simulink model "TITO_OC_2018"  (Simulink 9.1)
settings: Solver=ode45  StartTime=0.0  StopTime=100  RelTol=1e-3  EnableMultiTasking=on
undefined symbols (not defined in the file): T0
libraries: simulink x4
settings Model: Creator=petr  LastModifiedBy=NICHOLAS ANG
settings DataIOCC: LimitDataPoints=on  SignalLoggingSaveFormat=ModelDataLogs
settings OptimizationCC: ExpressionDepthLimit=2147483647  InitFltsAndDblsToZero=on
settings DebuggingCC: SolverPrmCheckMsg=warning  FcnCallInpInsideContextMsg=warning  StateNameClashWarn=warning

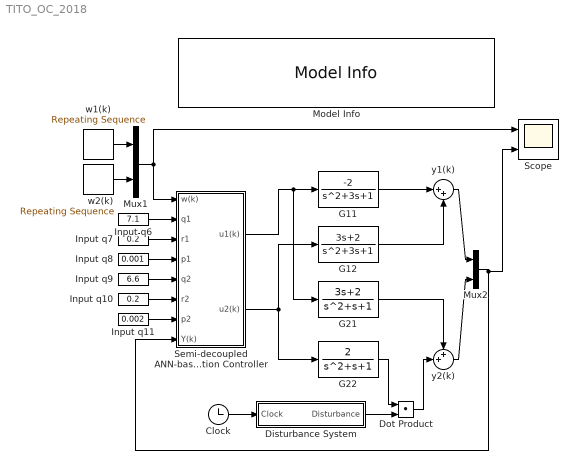
== system TITO_OC_2018 ==
  Clock : Clock
  Disturbance System : Subsystem
  Dot Product : DotProduct  InputSameDT=on  OutDataTypeStr=Inherit: Inherit via internal rule
  G11 : TransferFcn  Numerator=[-2]  Denominator=[1 3 1]
  G12 : TransferFcn  Numerator=[3 2]  Denominator=[1 3 1]
  G21 : TransferFcn  Numerator=[3 2]  Denominator=[1 1 1]
  G22 : TransferFcn  Numerator=[2]  Denominator=[1 1 1]
  Input q10 : Constant  Value=0.2
  Input q11 : Constant  Value=0.002
  Input q6 : Constant  Value=7.1
  Input q7 : Constant  Value=0.2
  Input q8 : Constant  Value=0.001
  Input q9 : Constant  Value=6.6
  Model Info : simulink/Model-Wide Utilities/Model Info  Frame=on  DisplayStringWithTags=|  HorizontalTextAlignment=Left  LeftAlignmentValue=0.02
      | "A Proposed TITO Self-tuning Control Scheme"
      | 
      | Designers: Guang Jun Nicholas Ang, Wei Ze Lim, Choo Min Lim
      | Created: August 2017
      | Revised: 19 June 2018
  Mux1 : Mux  Inputs=2
  Mux2 : Mux  Inputs=2
  "Scope  " : Scope  NumInputPorts=2
  Semi-decoupled ANN-based Optimization Controller : Subsystem
  w1(k) : simulink/Sources/Repeating Sequence  rep_seq_t=20*[0 0.4999 0.5 1.4999]  rep_seq_y=[1 1 2 2]
  w2(k) : simulink/Sources/Repeating Sequence  rep_seq_t=20*[0 0.9999 1.0 1.4999]  rep_seq_y=0.52*[1 1 2 2]
  y1(k) : Sum  Inputs=|++
  y2(k) : Sum  Inputs=++|
  wires:
  G12/1 -> y1(k)/2
  G21/1 -> y2(k)/1
  y2(k)/1 -> Mux2/2
  Input q6/1 -> Semi-decoupled ANN-based Optimization Controller/2(q1)
  Input q7/1 -> Semi-decoupled ANN-based Optimization Controller/3(r1)
  Input q8/1 -> Semi-decoupled ANN-based Optimization Controller/4(p1)
  Input q9/1 -> Semi-decoupled ANN-based Optimization Controller/5(q2)
  Input q10/1 -> Semi-decoupled ANN-based Optimization Controller/6(r2)
  Input q11/1 -> Semi-decoupled ANN-based Optimization Controller/7(p2)
  Semi-decoupled ANN-based Optimization Controller/1("u1(k)  ") -> G11/1, G21/1
  Semi-decoupled ANN-based Optimization Controller/2("u2(k) ") -> G22/1, G12/1
  Mux2/1 -> "Scope  "/2, Semi-decoupled ANN-based Optimization Controller/8(Y(k))
  w2(k)/1 -> Mux1/2
  Mux1/1 -> "Scope  "/1, Semi-decoupled ANN-based Optimization Controller/1(w(k))
  y1(k)/1 -> Mux2/1
  G11/1 -> y1(k)/1
  Disturbance System/1(Disturbance) -> Dot Product/2
  G22/1 -> Dot Product/1
  Dot Product/1 -> y2(k)/2
  Clock/1 -> Disturbance System/1(Clock)
  w1(k)/1 -> Mux1/1

== system TITO_OC_2018/Disturbance System ==
  Clock : Inport
  Compare To Constant : simulink/Logic and Bit Operations/Compare To Constant  relop=>=  const=45  OutDataTypeStr=boolean
  Constant : Constant
  Constant1 : Constant  Value=1.25
  Display6 : Display
  Switch : Switch  Criteria=u2 > Threshold  Threshold=159
  Disturbance : Outport
  wires:
  Compare To Constant/1 -> Switch/2
  Constant/1 -> Switch/3
  Constant1/1 -> Switch/1
  Switch/1 -> Disturbance/1, Display6/1
  Clock/1 -> Compare To Constant/1

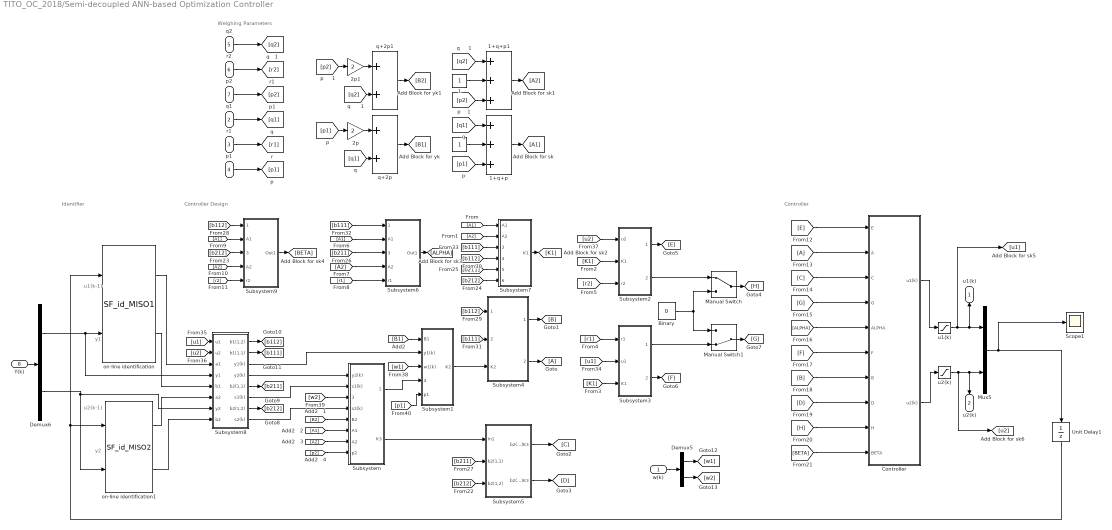
== system TITO_OC_2018/Semi-decoupled ANN-based Optimization Controller ==
  note: Weighing Parameters
  note: y2
  note: Controller
  note: u2(k-1)
  note: y1
  note: u1(k-1)
  note: Controller Design
  note: Identifier
  w(k) : Inport
  q1 : Inport  Port=2
  r1 : Inport  Port=3
  p1 : Inport  Port=4
  q2 : Inport  Port=5
  r2 : Inport  Port=6
  p2 : Inport  Port=7
  Y(k) : Inport  Port=8
  "      " : Constant
  "      1" : Constant
  1+q+p : Sum  Inputs=+++
  1+q+p1 : Sum  Inputs=+++
  2p : Gain  Gain=2
  2p1 : Gain  Gain=2
  Binary : Constant  Value=0
  Controller : Subsystem
  Demux5 : Demux  Outputs=2
  Demux6 : Demux  Outputs=2
  Manual Switch : ManualSwitch
  Manual Switch1 : ManualSwitch  CurrentSetting=0
  Mux5 : Mux  Inputs=2
  Scope1 : Scope
  Subsystem : Subsystem
  Subsystem1 : Subsystem
  Subsystem2 : Subsystem
  Subsystem3 : Subsystem
  Subsystem4 : Subsystem
  Subsystem5 : Subsystem
  Subsystem6 : Subsystem
  Subsystem7 : Subsystem
  Subsystem8 : Subsystem
  Subsystem9 : Subsystem
  Unit Delay1 : UnitDelay  SampleTime=T0
  on-line identification : M-S-Function  FunctionName=SF_id_MISO1  Parameters=T01, model_type1, id_alg1, ni, na1, nb1, nc1, origin_pass1, Theta01, C01, phi01, lam01, nu01, rho1
  on-line identification1 : M-S-Function  FunctionName=SF_id_MISO2  Parameters=T02, model_type2, id_alg2, ni, na2, nb2, nc2, origin_pass2, Theta02, C02, phi02, lam02, nu02, rho2
  q+2p : Sum
  q+2p1 : Sum
  u1(k) : Saturate  UpperLimit=1  LowerLimit=-1
  u2(k) : Saturate  UpperLimit=1  LowerLimit=0
  "u1(k)  " : Outport
  "u2(k) " : Outport  Port=2
  wires:
  Demux6/2 -> Subsystem8/7(y2), on-line identification1/2
  Demux6/1 -> Subsystem8/4(y1), on-line identification/2
  Unit Delay1/1 -> on-line identification/1, on-line identification1/1
  Y(k)/1 -> Demux6/1
  Controller/1(u1(k)) -> u1(k)/1
  Controller/2(u2(k)) -> u2(k)/1
  [E] -> Controller/1(E)
  [A] -> Controller/2(A)
  [C] -> Controller/3(C)
  [G] -> Controller/4(G)
  [ALPHA] -> Controller/5(ALPHA)
  [F] -> Controller/6(F)
  [B] -> Controller/7(B)
  [D] -> Controller/8(D)
  [H] -> Controller/9(H)
  [BETA] -> Controller/10(BETA)
  1+q+p1/1 -> [A2]
  q+2p1/1 -> [B2]
  1+q+p/1 -> [A1]
  q+2p/1 -> [B1]
  q2/1 -> [q2]
  [p2] -> 2p1/1
  [p1] -> 2p/1
  [q2] -> 1+q+p1/1
  "      1"/1 -> 1+q+p1/2
  [p2] -> 1+q+p1/3
  2p/1 -> q+2p/1
  "      "/1 -> 1+q+p/2
  [q1] -> 1+q+p/1
  p2/1 -> [p2]
  r2/1 -> [r2]
  2p1/1 -> q+2p1/1
  [q1] -> q+2p/2
  [q2] -> q+2p1/2
  q1/1 -> [q1]
  [p1] -> 1+q+p/3
  r1/1 -> [r1]
  p1/1 -> [p1]
  Subsystem8/1(b1(1,2)) -> [b112]
  Subsystem8/2(b1(1,1)) -> [b111]
  Subsystem8/5(b2(1,1)) -> [b211]
  Subsystem8/7(b2(1,2)) -> [b212]
  on-line identification/1 -> Subsystem8/3(a1)
  on-line identification/2 -> Subsystem8/5(b1)
  Subsystem8/4(y2(k)) -> Subsystem/1(y2(k))
  Subsystem8/6(s1(k)) -> Subsystem/2(s1(k))
  Subsystem8/8(s2(k)) -> Subsystem/4(s2(k))
  [B2] -> Subsystem/5(B2)
  [A1] -> Subsystem/6(A1)
  [A2] -> Subsystem/7(A2)
  [B1] -> Subsystem1/1(B1)
  Subsystem8/3(y1(k)) -> Subsystem1/2(y1(k))
  [w1] -> Subsystem1/3(w1(k))
  Subsystem/1(A1s1(k)) -> Subsystem1/4(A1s1(k))
  [K1] -> Subsystem2/2(K1)
  [r2] -> Subsystem2/3(r2)
  Subsystem2/1(K1u2(k)) -> [E]
  [r1] -> Subsystem3/1(r1)
  [K1] -> Subsystem3/3(K1)
  Subsystem3/2(K1u1(k)) -> [F]
  Subsystem1/1(K2) -> Subsystem4/3(K2)
  Subsystem4/1(b1(1,2)K2) -> [B]
  Subsystem4/2(b1(1,1)K2) -> [A]
  Subsystem/2(K3) -> Subsystem5/1(In1)
  Subsystem5/1(b2(1,1)K3) -> [C]
  Subsystem5/2(b2(1,2)K3) -> [D]
  [A1] -> Subsystem6/2(A1)
  [A2] -> Subsystem6/4(A2)
  [r1] -> Subsystem6/5(r1)
  Subsystem6/1(Out1) -> [ALPHA]
  [A1] -> Subsystem7/1(A1)
  [A2] -> Subsystem7/2(A2)
  Subsystem7/1(K1) -> [K1]
  [A1] -> Subsystem9/2(A1)
  [A2] -> Subsystem9/4(A2)
  [r2] -> Subsystem9/5(r2)
  Subsystem9/1(Out1) -> [BETA]
  u2(k)/1 -> [u2], "u2(k) "/1, Mux5/2
  Mux5/1 -> Scope1/1, Unit Delay1/1
  on-line identification1/1 -> Subsystem8/6(a2)
  on-line identification1/2 -> Subsystem8/8(b2)
  [b212] -> Subsystem5/3(b2(1,2))
  [b212] -> Subsystem9/3(b2(1,2))
  [b212] -> Subsystem7/6(b2(1,2))
  [b211] -> Subsystem7/5(b2(1,1))
  [b211] -> Subsystem6/3(b2(1,1))
  [b211] -> Subsystem5/2(b2(1,1))
  [b112] -> Subsystem9/1(b1(1,2))
  [b112] -> Subsystem4/1(b1(1,2))
  [b112] -> Subsystem7/4(b1(1,2))
  [b111] -> Subsystem4/2(b1(1,1))
  [b111] -> Subsystem6/1(b1(1,1))
  [b111] -> Subsystem7/3(b1(1,1))
  u1(k)/1 -> [u1], "u1(k)  "/1, Mux5/1
  [u1] -> Subsystem3/2(u1)
  [u1] -> Subsystem8/1(u1)
  [u2] -> Subsystem8/2(u2)
  [u2] -> Subsystem2/1(u2)
  w(k)/1 -> Demux5/1
  Demux5/1 -> [w1]
  Demux5/2 -> [w2]
  [w2] -> Subsystem/3(w2(k))
  Binary/1 -> Manual Switch1/1, Manual Switch/2
  Manual Switch1/1 -> [G]
  Subsystem3/1(r1u1(k-1)) -> Manual Switch1/2
  Subsystem2/2(r2u2(k-1)) -> Manual Switch/1
  Manual Switch/1 -> [H]
  [p2] -> Subsystem/8(p2)
  [p1] -> Subsystem1/5(p1)

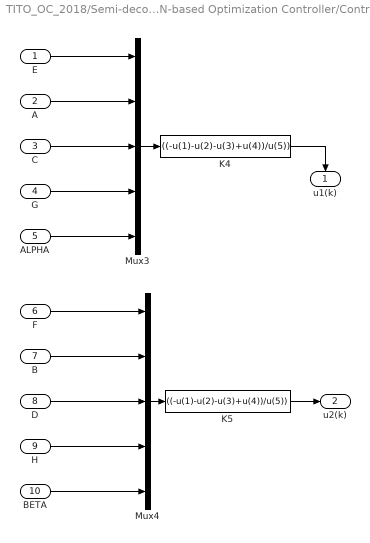
== system TITO_OC_2018/Semi-decoupled ANN-based Optimization Controller/Controller ==
  E : Inport
  A : Inport  Port=2
  C : Inport  Port=3
  G : Inport  Port=4
  ALPHA : Inport  Port=5
  F : Inport  Port=6
  B : Inport  Port=7
  D : Inport  Port=8
  H : Inport  Port=9
  BETA : Inport  Port=10
  K4 : Fcn  Expr=((-u(1)-u(2)-u(3)+u(4))/u(5))
  K5 : Fcn  Expr=((-u(1)-u(2)-u(3)+u(4))/u(5))
  Mux3 : Mux  Inputs=5
  Mux4 : Mux  Inputs=5
  u1(k) : Outport
  u2(k) : Outport  Port=2
  wires:
  B/1 -> Mux4/2
  K5/1 -> u2(k)/1
  Mux4/1 -> K5/1
  E/1 -> Mux3/1
  ALPHA/1 -> Mux3/5
  F/1 -> Mux4/1
  BETA/1 -> Mux4/5
  C/1 -> Mux3/3
  K4/1 -> u1(k)/1
  A/1 -> Mux3/2
  Mux3/1 -> K4/1
  H/1 -> Mux4/4
  G/1 -> Mux3/4
  D/1 -> Mux4/3

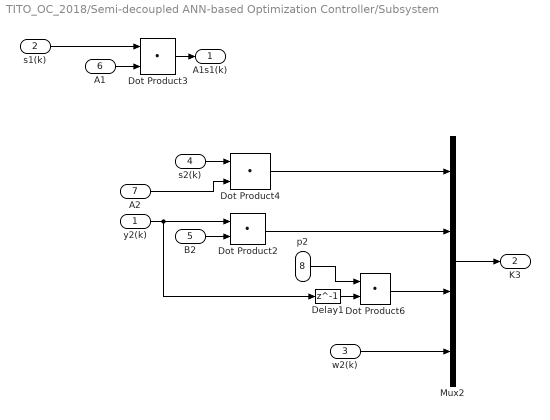
== system TITO_OC_2018/Semi-decoupled ANN-based Optimization Controller/Subsystem ==
  y2(k) : Inport
  s1(k) : Inport  Port=2
  w2(k) : Inport  Port=3
  s2(k) : Inport  Port=4
  B2 : Inport  Port=5
  A1 : Inport  Port=6
  A2 : Inport  Port=7
  p2 : Inport  Port=8
  Delay1 : Delay  DelayLength=1  SampleTime=T0
  Dot Product{2..4,6} (4 alike) : DotProduct  InputSameDT=on  OutDataTypeStr=Inherit: Inherit via internal rule
  Mux2 : Mux
  A1s1(k) : Outport
  K3 : Outport  Port=2
  wires:
  Dot Product2/1 -> Mux2/2
  Dot Product3/1 -> A1s1(k)/1
  Dot Product6/1 -> Mux2/3
  A2/1 -> Dot Product4/2
  B2/1 -> Dot Product2/2
  p2/1 -> Dot Product6/1
  Mux2/1 -> K3/1
  A1/1 -> Dot Product3/2
  Dot Product4/1 -> Mux2/1
  Delay1/1 -> Dot Product6/2
  w2(k)/1 -> Mux2/4
  y2(k)/1 -> Delay1/1, Dot Product2/1
  s1(k)/1 -> Dot Product3/1
  s2(k)/1 -> Dot Product4/1

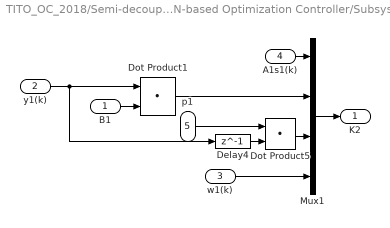
== system TITO_OC_2018/Semi-decoupled ANN-based Optimization Controller/Subsystem1 ==
  B1 : Inport
  y1(k) : Inport  Port=2
  w1(k) : Inport  Port=3
  A1s1(k) : Inport  Port=4
  p1 : Inport  Port=5
  Delay4 : Delay  DelayLength=1  SampleTime=T0
  Dot Product1 : DotProduct  InputSameDT=on  OutDataTypeStr=Inherit: Inherit via internal rule
  Dot Product5 : DotProduct  InputSameDT=on  OutDataTypeStr=Inherit: Inherit via internal rule
  Mux1 : Mux
  K2 : Outport
  wires:
  B1/1 -> Dot Product1/2
  p1/1 -> Dot Product5/1
  Dot Product5/1 -> Mux1/3
  Dot Product1/1 -> Mux1/2
  Delay4/1 -> Dot Product5/2
  w1(k)/1 -> Mux1/4
  Mux1/1 -> K2/1
  A1s1(k)/1 -> Mux1/1
  y1(k)/1 -> Delay4/1, Dot Product1/1

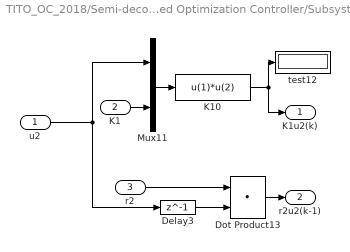
== system TITO_OC_2018/Semi-decoupled ANN-based Optimization Controller/Subsystem2 ==
  u2 : Inport
  K1 : Inport  Port=2
  r2 : Inport  Port=3
  Delay3 : Delay  DelayLength=1  SampleTime=T0
  Dot Product13 : DotProduct  InputSameDT=on  OutDataTypeStr=Inherit: Inherit via internal rule
  K10 : Fcn  Expr=u(1)*u(2)
  Mux11 : Mux  Inputs=2
  test12 : Display
  K1u2(k) : Outport
  r2u2(k-1) : Outport  Port=2
  wires:
  Delay3/1 -> Dot Product13/2
  r2/1 -> Dot Product13/1
  K1/1 -> Mux11/2
  Mux11/1 -> K10/1
  K10/1 -> K1u2(k)/1, test12/1
  Dot Product13/1 -> r2u2(k-1)/1
  u2/1 -> Mux11/1, Delay3/1

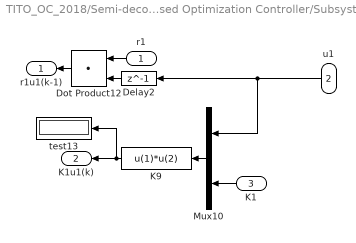
== system TITO_OC_2018/Semi-decoupled ANN-based Optimization Controller/Subsystem3 ==
  r1 : Inport
  u1 : Inport  Port=2
  K1 : Inport  Port=3
  Delay2 : Delay  DelayLength=1  SampleTime=T0
  Dot Product12 : DotProduct  InputSameDT=on  OutDataTypeStr=Inherit: Inherit via internal rule
  K9 : Fcn  Expr=u(1)*u(2)
  Mux10 : Mux  Inputs=2
  test13 : Display
  r1u1(k-1) : Outport
  K1u1(k) : Outport  Port=2
  wires:
  u1/1 -> Mux10/1, Delay2/1
  Delay2/1 -> Dot Product12/2
  r1/1 -> Dot Product12/1
  K1/1 -> Mux10/2
  Dot Product12/1 -> r1u1(k-1)/1
  K9/1 -> K1u1(k)/1, test13/1
  Mux10/1 -> K9/1

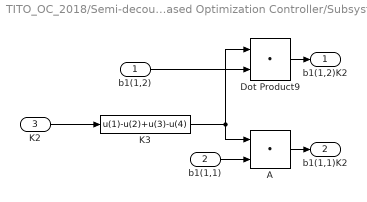
== system TITO_OC_2018/Semi-decoupled ANN-based Optimization Controller/Subsystem4 ==
  b1(1,2) : Inport
  b1(1,1) : Inport  Port=2
  K2 : Inport  Port=3
  A : DotProduct  InputSameDT=on  OutDataTypeStr=Inherit: Inherit via internal rule
  Dot Product9 : DotProduct  InputSameDT=on  OutDataTypeStr=Inherit: Inherit via internal rule
  K3 : Fcn  Expr=u(1)-u(2)+u(3)-u(4)
  b1(1,2)K2 : Outport
  b1(1,1)K2 : Outport  Port=2
  wires:
  b1(1,2)/1 -> Dot Product9/2
  b1(1,1)/1 -> A/2
  A/1 -> b1(1,1)K2/1
  K3/1 -> A/1, Dot Product9/1
  Dot Product9/1 -> b1(1,2)K2/1
  K2/1 -> K3/1

== system TITO_OC_2018/Semi-decoupled ANN-based Optimization Controller/Subsystem5 ==
  note: D
  note: C
  In1 : Inport
  b2(1,1) : Inport  Port=2
  b2(1,2) : Inport  Port=3
  Dot Product10 : DotProduct  InputSameDT=on  OutDataTypeStr=Inherit: Inherit via internal rule
  Dot Product8 : DotProduct  InputSameDT=on  OutDataTypeStr=Inherit: Inherit via internal rule
  K1 : Fcn  Expr=u(1)-u(2)+u(3)-u(4)
  b2(1,1)K3 : Outport
  b2(1,2)K3 : Outport  Port=2
  wires:
  b2(1,1)/1 -> Dot Product8/2
  b2(1,2)/1 -> Dot Product10/2
  Dot Product8/1 -> b2(1,1)K3/1
  Dot Product10/1 -> b2(1,2)K3/1
  K1/1 -> Dot Product10/1, Dot Product8/1
  In1/1 -> K1/1

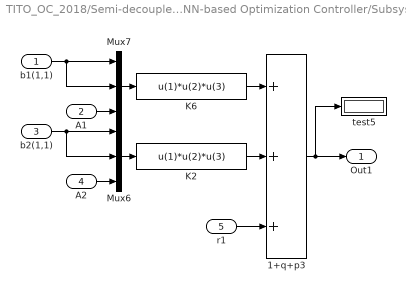
== system TITO_OC_2018/Semi-decoupled ANN-based Optimization Controller/Subsystem6 ==
  b1(1,1) : Inport
  A1 : Inport  Port=2
  b2(1,1) : Inport  Port=3
  A2 : Inport  Port=4
  r1 : Inport  Port=5
  1+q+p3 : Sum  Inputs=+++
  K2 : Fcn  Expr=u(1)*u(2)*u(3)
  K6 : Fcn  Expr=u(1)*u(2)*u(3)
  Mux6 : Mux  Inputs=3
  Mux7 : Mux  Inputs=3
  test5 : Display
  Out1 : Outport
  wires:
  b1(1,1)/1 -> Mux7/2, Mux7/1
  b2(1,1)/1 -> Mux6/1, Mux6/2
  A2/1 -> Mux6/3
  1+q+p3/1 -> Out1/1, test5/1
  K6/1 -> 1+q+p3/1
  A1/1 -> Mux7/3
  K2/1 -> 1+q+p3/2
  r1/1 -> 1+q+p3/3
  Mux6/1 -> K2/1
  Mux7/1 -> K6/1

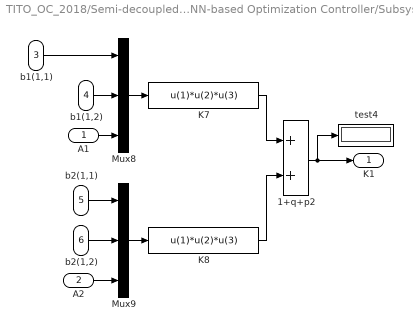
== system TITO_OC_2018/Semi-decoupled ANN-based Optimization Controller/Subsystem7 ==
  A1 : Inport
  A2 : Inport  Port=2
  b1(1,1) : Inport  Port=3
  b1(1,2) : Inport  Port=4
  b2(1,1) : Inport  Port=5
  b2(1,2) : Inport  Port=6
  1+q+p2 : Sum
  K7 : Fcn  Expr=u(1)*u(2)*u(3)
  K8 : Fcn  Expr=u(1)*u(2)*u(3)
  Mux8 : Mux  Inputs=3
  Mux9 : Mux  Inputs=3
  test4 : Display
  K1 : Outport
  wires:
  1+q+p2/1 -> test4/1, K1/1
  A1/1 -> Mux8/3
  Mux8/1 -> K7/1
  K8/1 -> 1+q+p2/2
  A2/1 -> Mux9/3
  K7/1 -> 1+q+p2/1
  Mux9/1 -> K8/1
  b1(1,1)/1 -> Mux8/1
  b2(1,1)/1 -> Mux9/1
  b2(1,2)/1 -> Mux9/2
  b1(1,2)/1 -> Mux8/2

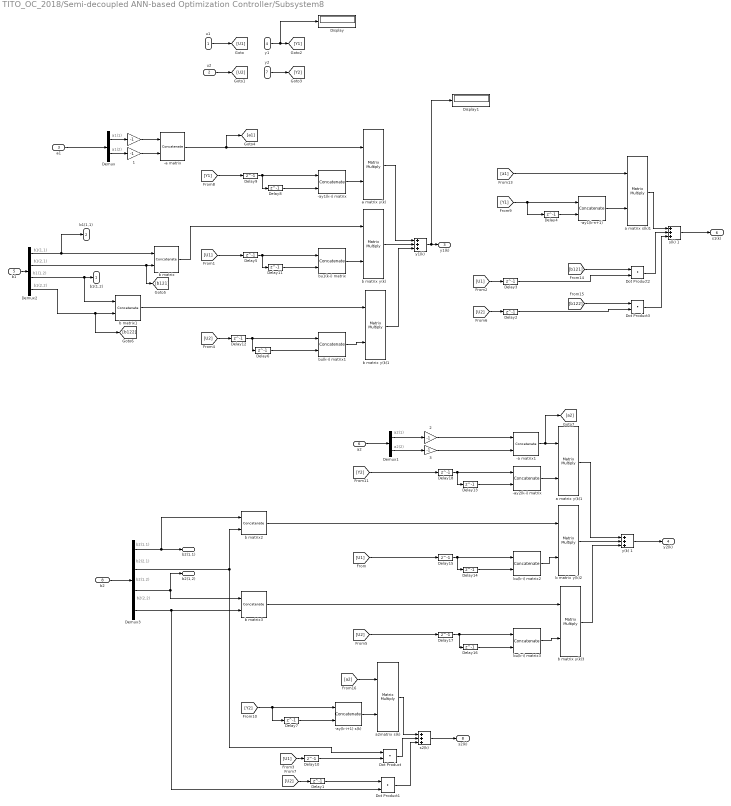
== system TITO_OC_2018/Semi-decoupled ANN-based Optimization Controller/Subsystem8 ==
  note: b1(1,1)
  note: b1(2,1)
  note: b1(1,2)
  note: b1(2,2)
  note: a2(1)
  note: a2(2)
  note: b2(1,1)
  note: b2(2,1)
  note: b2(1,2)
  note: b2(2,2)
  note: a1(1)
  note: a1(2)
  u1 : Inport
  u2 : Inport  Port=2
  a1 : Inport  Port=3
  y1 : Inport  Port=4
  b1 : Inport  Port=5
  a2 : Inport  Port=6
  y2 : Inport  Port=7
  b2 : Inport  Port=8
     {,1..3} (4 alike) : Gain  Gain=-1
  -a matrix : Concatenate  Mode=Multidimensional array  ConcatenateDimension=2
  -a matrix1 : Concatenate  Mode=Multidimensional array  ConcatenateDimension=2
  -ay(k-i+1) s(k) : Concatenate  Mode=Multidimensional array
  -ay1(k-i) matrix : Concatenate  Mode=Multidimensional array
  -ay1(k-n+1) : Concatenate  Mode=Multidimensional array
  -ay2(k-i) matrix : Concatenate  Mode=Multidimensional array
  Delay{1..18} (18 alike) : Delay  DelayLength=1  SampleTime=T0
  Demux : Demux  Outputs=2
  Demux1 : Demux  Outputs=2
  Demux2 : Demux
  Demux3 : Demux
  Display : Display
  Display1 : Display
  Dot Product{,1..3} (4 alike) : DotProduct  InputSameDT=on  OutDataTypeStr=Inherit: Inherit via internal rule
  a matrix s(k)1 : Product  Multiplication=Matrix(*)
  a matrix y(k) : Product  Multiplication=Matrix(*)
  a matrix y(k)1 : Product  Multiplication=Matrix(*)
  a2matrix s(k) : Product  Multiplication=Matrix(*)
  b matrix{,1..3} (4 alike) : Concatenate  Mode=Multidimensional array  ConcatenateDimension=2
  b matrix y(k){,1..3} (4 alike) : Product  Multiplication=Matrix(*)
  bu(k-i) matrix1 : Concatenate  Mode=Multidimensional array
  bu(k-i) matrix2 : Concatenate  Mode=Multidimensional array
  bu(k-i) matrix3 : Concatenate  Mode=Multidimensional array
  bu1(k-i) matrix : Concatenate  Mode=Multidimensional array
  s(k) 1 : Sum  Inputs=+++
  "s2(k) " : Sum  Inputs=+++
  y(k) 1 : Sum  Inputs=+++
  "y1(k) " : Sum  Inputs=+++
  b1(1,2) : Outport
  b1(1,1) : Outport  Port=2
  y1(k) : Outport  Port=3
  y2(k) : Outport  Port=4
  b2(1,1) : Outport  Port=5
  s1(k) : Outport  Port=6
  b2(1,2) : Outport  Port=7
  s2(k) : Outport  Port=8
  wires:
  Demux2/3 -> b matrix1/1, b1(1,2)/1
  y(k) 1/1 -> y2(k)/1
  "y1(k) "/1 -> Display1/1, y1(k)/1
  s(k) 1/1 -> s1(k)/1
  "s2(k) "/1 -> s2(k)/1
  Demux3/1 -> b matrix2/1, b2(1,1)/1
  b1/1 -> Demux2/1
  Demux2/1 -> b1(1,1)/1, b matrix/1
  "   2"/1 -> -a matrix1/1
  Demux1/1 -> "   2"/1
  Demux1/2 -> "   3"/1
  "   3"/1 -> -a matrix1/2
  a2/1 -> Demux1/1
  b2/1 -> Demux3/1
  Dot Product1/1 -> "s2(k) "/3
  -ay(k-i+1) s(k)/1 -> a2matrix s(k)/2
  Demux3/2 -> b matrix2/2, Dot Product/1
  Delay7/1 -> -ay(k-i+1) s(k)/2
  Dot Product/1 -> "s2(k) "/2
  a2matrix s(k)/1 -> "s2(k) "/1
  "   "/1 -> -a matrix/1
  Demux/2 -> "   1"/1
  "   1"/1 -> -a matrix/2
  Demux/1 -> "   "/1
  a1/1 -> Demux/1
  Dot Product3/1 -> s(k) 1/3
  u2/1 -> [U2]
  Demux2/4 -> [b122], b matrix1/2
  u1/1 -> [U1]
  -ay1(k-n+1)/1 -> a matrix s(k)1/2
  Demux2/2 -> [b121], b matrix/2
  Delay4/1 -> -ay1(k-n+1)/2
  Dot Product2/1 -> s(k) 1/2
  a matrix s(k)1/1 -> s(k) 1/1
  [U1] -> Delay3/1
  [U1] -> Delay10/1
  [U2] -> Delay2/1
  [U2] -> Delay1/1
  [Y1] -> Delay4/1, -ay1(k-n+1)/1
  y2/1 -> [Y2]
  [Y2] -> Delay7/1, -ay(k-i+1) s(k)/1
  Delay6/1 -> bu(k-i) matrix1/2
  bu(k-i) matrix1/1 -> b matrix y(k)1/2
  Delay12/1 -> bu(k-i) matrix1/1, Delay6/1
  b matrix y(k)1/1 -> "y1(k) "/3
  [U2] -> Delay12/1
  b matrix1/1 -> b matrix y(k)1/1
  Delay11/1 -> bu1(k-i) matrix/2
  a matrix y(k)/1 -> "y1(k) "/1
  -ay1(k-i) matrix/1 -> a matrix y(k)/2
  bu1(k-i) matrix/1 -> b matrix y(k)/2
  Delay5/1 -> bu1(k-i) matrix/1, Delay11/1
  Delay8/1 -> -ay1(k-i) matrix/2
  Delay9/1 -> Delay8/1, -ay1(k-i) matrix/1
  b matrix y(k)/1 -> "y1(k) "/2
  [U1] -> Delay5/1
  b matrix/1 -> b matrix y(k)/1
  [Y1] -> Delay9/1
  Delay16/1 -> bu(k-i) matrix3/2
  bu(k-i) matrix3/1 -> b matrix y(k)3/2
  Delay17/1 -> bu(k-i) matrix3/1, Delay16/1
  b matrix y(k)3/1 -> y(k) 1/3
  [U2] -> Delay17/1
  b matrix3/1 -> b matrix y(k)3/1
  Delay14/1 -> bu(k-i) matrix2/2
  a matrix y(k)1/1 -> y(k) 1/1
  -ay2(k-i) matrix/1 -> a matrix y(k)1/2
  bu(k-i) matrix2/1 -> b matrix y(k)2/2
  Delay15/1 -> Delay14/1, bu(k-i) matrix2/1
  Delay13/1 -> -ay2(k-i) matrix/2
  Delay18/1 -> Delay13/1, -ay2(k-i) matrix/1
  b matrix y(k)2/1 -> y(k) 1/2
  [U1] -> Delay15/1
  -a matrix1/1 -> [a2], a matrix y(k)1/1
  b matrix2/1 -> b matrix y(k)2/1
  [Y2] -> Delay18/1
  -a matrix/1 -> a matrix y(k)/1, [a1]
  [a1] -> a matrix s(k)1/1
  [b121] -> Dot Product2/1
  [b122] -> Dot Product3/1
  [a2] -> a2matrix s(k)/1
  Demux3/3 -> b2(1,2)/1, b matrix3/1
  Delay10/1 -> Dot Product/2
  Delay1/1 -> Dot Product1/1
  Demux3/4 -> Dot Product1/2, b matrix3/2
  Delay2/1 -> Dot Product3/2
  Delay3/1 -> Dot Product2/2
  y1/1 -> Display/1, [Y1]

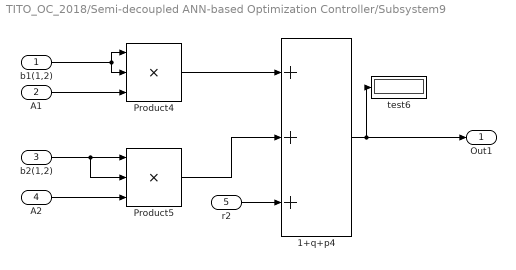
== system TITO_OC_2018/Semi-decoupled ANN-based Optimization Controller/Subsystem9 ==
  b1(1,2) : Inport
  A1 : Inport  Port=2
  b2(1,2) : Inport  Port=3
  A2 : Inport  Port=4
  r2 : Inport  Port=5
  1+q+p4 : Sum  Inputs=+++
  Product4 : Product  Inputs=3
  Product5 : Product  Inputs=3
  test6 : Display
  Out1 : Outport
  wires:
  r2/1 -> 1+q+p4/3
  A1/1 -> Product4/3
  Product5/1 -> 1+q+p4/2
  1+q+p4/1 -> test6/1, Out1/1
  Product4/1 -> 1+q+p4/1
  A2/1 -> Product5/3
  b1(1,2)/1 -> Product4/1, Product4/2
  b2(1,2)/1 -> Product5/2, Product5/1
